simulink model "Houghline_real_nocolor"  (R2016a)
settings: Solver=VariableStepAuto  StartTime=0.0  StopTime=inf  RelTol=1e-3
undefined symbols (not defined in the file): gray, Rec, SDTV
libraries: visionconversions x4, visiontransforms x3, visionfilter x2, visiontextngfix x2, dspvision x1, visionanalysis x1, visionstatistics x1
settings Model: Creator=Yewly  LastModifiedBy=Yewly
settings GRTTargetCC: GeneratePreprocessorConditionals=Use local settings

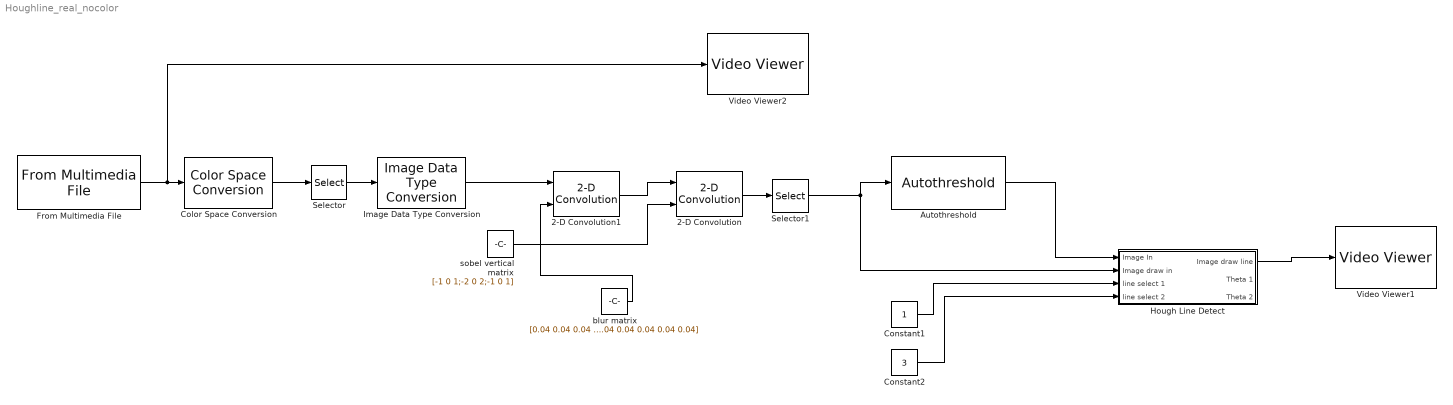
== system Houghline_real_nocolor ==
  2-D Convolution : visionfilter/2-D Convolution  outSize=Full  normalize=off  outputMode=Binary point scaling  outputWordLength=32  outputFracLength=12  prodOutputMode=Binary point scaling  prodOutputWordLength=32  prodOutputFracLength=10  roundingMode=Floor  overflowMode=off
  2-D Convolution1 : visionfilter/2-D Convolution  outSize=Full  normalize=off  outputMode=Binary point scaling  outputWordLength=32  outputFracLength=12  prodOutputMode=Binary point scaling  prodOutputWordLength=32  prodOutputFracLength=10  roundingMode=Floor  overflowMode=off
  Autothreshold : visionconversions/Autothreshold  operator=>  threshOut=off  effMetricOut=off  userDefinedRange=off  umin=0  umax=255  outOfRngOpt=Warn and saturate  scaleThreshold=off  scaleFactor=1  P1Mode=Specify word length  P1WordLength=32  P1FracLength=30  P2Mode=Specify word length  P2WordLength=32  P2FracLength=22  P3Mode=Specify word length  P3WordLength=32  P3FracLength=14  P4Mode=Binary point scaling  P4WordLength=32  P4FracLength=15  Q1Mode=Specify word length  Q1WordLength=32  Q1FracLength=16  EMMode=Specify word length  EMWordLength=16  EMFracLength=14  roundingMode=Floor  overflowMode=off
  Color Space Conversion : visionconversions/Color Space  Conversion  conversion=Obsolete  conversionActive=R'G'B' to intensity  wp_str=D65  rec=Rec. 601 (SDTV)  sys=1125/60/2:1  imagePorts=One multidimensional signal
  Constant1 : Constant  OutDataTypeStr=double
  Constant2 : Constant  Value=3  OutDataTypeStr=double
  From Multimedia File : dspvision/From Multimedia File  inputFilename=lane2.mp4  loop=on  numPlays=inf  outputStreams=Video only  videoDataType=single  audioDataType=int16  inheritSampleTime=on  userDefinedSampleTime=1  noAudioOutput=off  isIntensityVideo=off  fourcc=RGB  colorVideoFormat=One multidimensional signal  outputEOF=off  dataOrg=Column-major  audioFrameSize=1024  computeAudioFrameSize=off  outSamplingMode=Sample based
  "Hough Line Detect " : Subsystem
  Image Data Type Conversion : visionconversions/Image Data Type Conversion  outDT=double  isSigned=on  wordLen=16  numFracBits=0
  Selector : Selector  NumberOfDimensions=2  InputPortWidth=3  IndexOptions=Starting index (dialog),Select all  Indices=220,1  OutputSizes=220,1
  Selector1 : Selector  NumberOfDimensions=2  InputPortWidth=3  IndexOptions=Starting index (dialog),Starting index (dialog)  Indices=10,10  OutputSizes=210,620
  Video Viewer1 : VideoViewer  colormapValue=gray(256)  FigPos=[720.2 362 526.4 247.2]
  Video Viewer2 : VideoViewer  colormapValue=gray(256)  FigPos=[367.4 844.4 714.4 445.6]
  blur matrix : Constant  Value=[0.04 0.04 0.04 0.04 0.04;0.04 0.04 0.04 0.04 0.04;0.04 0.04 0.04 0.04 0.04;0.04 0.04 0.04 0.04 0.04;0.04 0.04 0.04 0.04 0.04]  OutDataTypeStr=double
  sobel vertical matrix : Constant  Value=[-1 0 1;-2 0 2;-1 0 1]  OutDataTypeStr=double
  wires:
  "Hough Line Detect "/1("Image draw line ") -> Video Viewer1/1
  Constant1/1 -> "Hough Line Detect "/3(line select 1)
  Constant2/1 -> "Hough Line Detect "/4(line select 2)
  From Multimedia File/1 -> Video Viewer2/1, Color Space Conversion/1
  Color Space Conversion/1 -> Selector/1
  Autothreshold/1 -> "Hough Line Detect "/1(Image In)
  Selector/1 -> Image Data Type Conversion/1
  2-D Convolution/1 -> Selector1/1
  2-D Convolution1/1 -> 2-D Convolution/1
  Selector1/1 -> Autothreshold/1, "Hough Line Detect "/2("Image draw in ")
  Image Data Type Conversion/1 -> 2-D Convolution1/1
  blur matrix/1 -> 2-D Convolution1/2
  sobel vertical matrix/1 -> 2-D Convolution/2

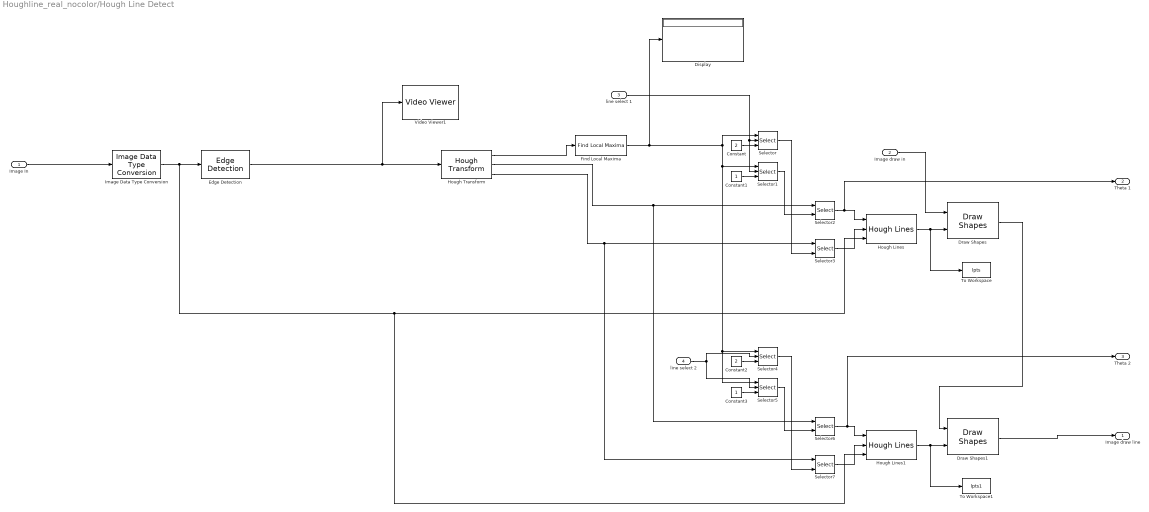
== system Houghline_real_nocolor/Hough Line Detect  ==
  Image In : Inport
  "Image draw in " : Inport  Port=2
  line select 1 : Inport  Port=3
  line select 2 : Inport  Port=4
  Constant : Constant  Value=2
  Constant1 : Constant
  Constant2 : Constant  Value=2
  Constant3 : Constant
  Display : Display
  Draw Shapes : visiontextngfix/Draw Shapes  shape=Lines  fill=off  lineWidth=10  fillClrSource=Specify via dialog  display=White  intensity=200  color=255  opacity=0.6  viewport=Entire image  antialiasing=off  inType=Obsolete  imagePorts=One multidimensional signal  prodOutputMode=Binary point scaling  prodOutputWordLength=32  prodOutputFracLength=14  memoryMode=Specify word length  memoryWordLength=16  memoryFracLength=14  roundingMode=Floor  overflowMode=off
  Draw Shapes1 : visiontextngfix/Draw Shapes  shape=Lines  fill=off  lineWidth=10  fillClrSource=Specify via dialog  display=White  intensity=200  color=255  opacity=0.6  viewport=Entire image  antialiasing=off  inType=Obsolete  imagePorts=One multidimensional signal  prodOutputMode=Binary point scaling  prodOutputWordLength=32  prodOutputFracLength=14  memoryMode=Specify word length  memoryWordLength=16  memoryFracLength=14  roundingMode=Floor  overflowMode=off
  Edge Detection : visionanalysis/Edge Detection  method=Sobel  outputType=Binary image  userDefinedThreshold=off  thresholdSource=Specify via dialog  threshold=20  thresholdTuning=4  edgeThinning=on  threshold_canny=[0.25 0.60]  autoPercent=70  sigma=1  prodOutputMode=Binary point scaling  prodOutputWordLength=32  prodOutputFracLength=8  roundingMode=Floor  overflowMode=off
  Find Local Maxima : visionstatistics/Find Local Maxima  num_peaks=100  nhood_size=[5 7]  src_thresh=Obsolete9b  src_thresh_inuse=Specify via dialog  threshold=10  inputIsHough=on  dt_peak=uint32  isOutVarDim=on  dt_count=uint32
  Hough Lines : visiontransforms/Hough Lines  sineCompMethod=Trigonometric function  thetaRes=pi/180  firstCoeffMode=Specify word length  firstCoeffWordLength=16  firstCoeffFracLength=15  prodOutputMode=Binary point scaling  prodOutputWordLength=32  prodOutputFracLength=16  roundingMode=Nearest  overflowMode=on
  Hough Lines1 : visiontransforms/Hough Lines  sineCompMethod=Trigonometric function  thetaRes=pi/180  firstCoeffMode=Specify word length  firstCoeffWordLength=16  firstCoeffFracLength=15  prodOutputMode=Binary point scaling  prodOutputWordLength=32  prodOutputFracLength=16  roundingMode=Nearest  overflowMode=on
  Hough Transform : visiontransforms/Hough Transform  theta_res=pi/360  rho_res=1  out_theta_rho=on  outdtmode=double  firstCoeffMode=Binary point scaling  firstCoeffWordLength=16  firstCoeffFracLength=14  secondCoeffMode=Binary point scaling  secondCoeffWordLength=32  secondCoeffFracLength=16  outputMode=Binary point scaling  outputWordLength=16  outputFracLength=0  accumMode=Binary point scaling  accumWordLength=32  accumFracLength=20  prodOutputMode=Binary point scaling  prodOutputWordLength=32  prodOutputFracLength=20  memoryMode=Binary point scaling  memoryWordLength=32  memoryFracLength=16  roundingMode=Nearest  overflowMode=on
  Image Data Type Conversion : visionconversions/Image Data Type Conversion  outDT=double  isSigned=on  wordLen=16  numFracBits=0
  Selector : Selector  NumberOfDimensions=2  InputPortWidth=2  IndexOptions=Index vector (port),Index vector (port)  Indices=1,1  OutputSizes=1,1
  Selector1 : Selector  NumberOfDimensions=2  InputPortWidth=2  IndexOptions=Starting index (port),Index vector (port)  Indices=1,1  OutputSizes=1,1
  Selector{2..3,6..7} (4 alike) : Selector  NumberOfDimensions=2  InputPortWidth=3  IndexOptions=Select all,Index vector (port)  Indices=[1 3],1  OutputSizes=1,1
  Selector4 : Selector  NumberOfDimensions=2  InputPortWidth=2  IndexOptions=Index vector (port),Index vector (port)  Indices=2,1  OutputSizes=1,1
  Selector5 : Selector  NumberOfDimensions=2  InputPortWidth=2  IndexOptions=Index vector (port),Index vector (port)  Indices=2,1  OutputSizes=1,1
  To Workspace : ToWorkspace  VariableName=lpts  SampleTime=-1
  To Workspace1 : ToWorkspace  VariableName=lpts1  SampleTime=-1
  Video Viewer1 : VideoViewer  colormapValue=gray(256)  FigPos=[154.6 360.4 563.2 241.6]
  "Image draw line " : Outport
  Theta 1 : Outport  Port=2
  Theta 2 : Outport  Port=3
  wires:
  Selector5/1 -> Selector6/2
  Draw Shapes1/1 -> "Image draw line "/1
  Constant1/1 -> Selector1/3
  Constant3/1 -> Selector5/3
  Selector3/1 -> Hough Lines/2
  Hough Transform/3 -> Selector7/1, Selector3/1
  Selector4/1 -> Selector7/2
  Hough Lines/1 -> To Workspace/1, Draw Shapes/2
  Hough Transform/1 -> Find Local Maxima/1
  Selector7/1 -> Hough Lines1/2
  Hough Lines1/1 -> To Workspace1/1, Draw Shapes1/2
  Selector1/1 -> Selector2/2
  Constant2/1 -> Selector4/3
  Selector/1 -> Selector3/2
  Draw Shapes/1 -> Draw Shapes1/1
  Selector2/1 -> Theta 1/1, Hough Lines/1
  Selector6/1 -> Theta 2/1, Hough Lines1/1
  line select 1/1 -> Selector1/2, Selector/2
  Constant/1 -> Selector/3
  line select 2/1 -> Selector5/2, Selector4/2
  Image Data Type Conversion/1 -> Hough Lines1/3, Hough Lines/3, Edge Detection/1
  Find Local Maxima/1 -> Display/1, Selector5/1, Selector4/1, Selector1/1, Selector/1
  Image In/1 -> Image Data Type Conversion/1
  "Image draw in "/1 -> Draw Shapes/1
  Hough Transform/2 -> Selector6/1, Selector2/1
  Edge Detection/1 -> Video Viewer1/1, Hough Transform/1
